simulink model "fxpdemo_lead_lag"  (Simulink 5.0)
settings: Solver=FixedStepDiscrete  SolverMode=SingleTasking  StartTime=0.0  StopTime=7.95  FixedStep=SampleTime  RelTol=1e-3  AbsTol=1e-6
PreLoadFcn:
  | preload_lead_lag
values from neighbouring files (symbols this model uses):
  PoleZ = 0.85    [preload_diff.m]
  SampleTime = 0.05    [preload_diff.m]    (also in preload_state_space.mat = 0.01)
undefined symbols (not defined in the file or in its folder): LagKdc, LagZeroZ, LeadKdc, LeadZeroZ
libraries: fixpt_lib_4 x8, fixpt_lib_3p1 x1
settings Model: CovMetricSettings=d  MinMaxOverflowLogging=MinMaxAndOverflow  Creator=andyb  LastModifiedBy=andyb  ExtModeTrigMode=oneshot  ExtModeArmWhenConnect=off  ExtModeAutoUpdateStatusClock=off  LimitDataPoints=off  IntegerOverflowMsg=none  ParameterDowncastMsg=warning  ParameterOverflowMsg=warning  ParameterPrecisionLossMsg=none  BooleanDataType=off

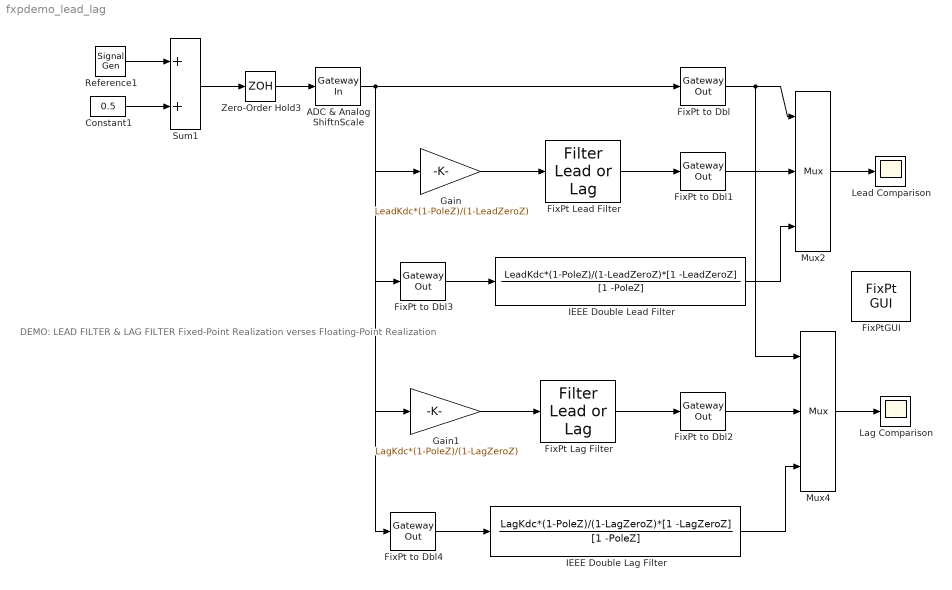
== system fxpdemo_lead_lag ==
  note: DEMO:
      |
      | LEAD FILTER
      | &
      | LAG FILTER
      |
      | Fixed-Point Realization
      | verses
      | Floating-Point Realization
  ADC & Analog ShiftnScale : fixpt_lib_4/Data Type/Gateway In  InRealWorld=Real World Value  OutputDataTypeScalingMode=Specify via dialog  OutDataType=sfix(8)  OutScaling=2^(-4)  RndMeth=Nearest  DoSatur=on
  Constant1 : Constant  Value=0.5
  FixPt Lag Filter : fixpt_lib_4/Filters/Filter Lead or Lag  PoleZ=PoleZ  ZeroZ=LagZeroZ  ICPrevOutput=0.0  ICPrevInput=0.0  DoSatur=off
  FixPt Lead Filter : fixpt_lib_4/Filters/Filter Lead or Lag  PoleZ=PoleZ  ZeroZ=LeadZeroZ  ICPrevOutput=0.0  ICPrevInput=0.0  DoSatur=off
  FixPt to Dbl{,1..4} (5 alike) : fixpt_lib_4/Data Type/Gateway Out  OutRealWorld=Real World Value  OutBuiltInType=double  DoSatur=off
  FixPtGUI : fixpt_lib_3p1/FixPt GUI
  Gain : Gain  Gain=LeadKdc*(1-PoleZ)/(1-LeadZeroZ)  ShowAdditionalParam=on  ParameterDataType=sfix( 16 )  ParameterScalingMode=Best Precision: Column-wise  ParameterScaling=2^-14  OutScaling=2^-10
  Gain1 : Gain  Gain=LagKdc*(1-PoleZ)/(1-LagZeroZ)  ShowAdditionalParam=on  ParameterDataType=sfix( 16 )  ParameterScalingMode=Best Precision: Column-wise  ParameterScaling=2^-14  OutScaling=2^-10
  IEEE Double Lag Filter : DiscreteFilter  Numerator=LagKdc*(1-PoleZ)/(1-LagZeroZ)*[1 -LagZeroZ]  Denominator=[1 -PoleZ]  SampleTime=SampleTime
  IEEE Double Lead Filter : DiscreteFilter  Numerator=LeadKdc*(1-PoleZ)/(1-LeadZeroZ)*[1 -LeadZeroZ]  Denominator=[1 -PoleZ]  SampleTime=SampleTime
  Lag Comparison : Scope
      settings: TickLabels=on  YMin=-3  YMax=4  SaveName=LagCompare
  Lead Comparison : Scope
      settings: TickLabels=on  TimeRange=8  YMin=-3  YMax=3  SaveName=LeadCompare
  Mux2 : Mux  Inputs=3
  Mux4 : Mux  Inputs=3
  Reference1 : SignalGenerator  WaveForm=square  Amplitude=-1.5  Frequency=1/8
  Sum1 : Sum  Inputs=2  SaturateOnIntegerOverflow=on  InputSameDT=on
  Zero-Order Hold3 : ZeroOrderHold  SampleTime=SampleTime
  wires:
  Reference1/1 -> Sum1/1
  Constant1/1 -> Sum1/2
  Zero-Order Hold3/1 -> ADC & Analog ShiftnScale/1
  Sum1/1 -> Zero-Order Hold3/1
  ADC & Analog ShiftnScale/1 -> FixPt to Dbl/1, FixPt to Dbl3/1, Gain/1, FixPt to Dbl4/1, Gain1/1
  FixPt to Dbl/1 -> Mux2/1, Mux4/1
  FixPt to Dbl1/1 -> Mux2/2
  IEEE Double Lead Filter/1 -> Mux2/3
  FixPt Lag Filter/1 -> FixPt to Dbl2/1
  IEEE Double Lag Filter/1 -> Mux4/3
  FixPt to Dbl4/1 -> IEEE Double Lag Filter/1
  FixPt to Dbl3/1 -> IEEE Double Lead Filter/1
  FixPt to Dbl2/1 -> Mux4/2
  Mux2/1 -> Lead Comparison/1
  Mux4/1 -> Lag Comparison/1
  FixPt Lead Filter/1 -> FixPt to Dbl1/1
  Gain/1 -> FixPt Lead Filter/1
  Gain1/1 -> FixPt Lag Filter/1
